simulink model "sampleModel1743_4_sub_sub"  (R2023a)
settings: Solver=VariableStepAuto  StartTime=0.0  StopTime=10.0  RelTol=1e-3
libraries: hdlsllib x4, simulink x2
settings Model: Creator=user1  LastModifiedBy=user1

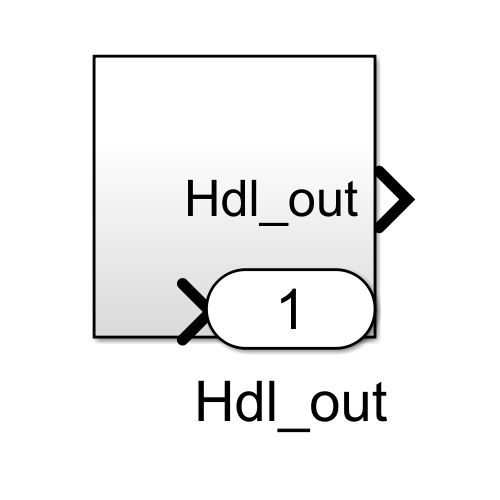
[thumbnail: Simulink's stored preview of the top-level diagram]
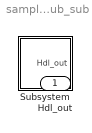
== system sampleModel1743_4_sub_sub ==
  Subsystem : Subsystem
  Hdl_out : Outport  OutDataTypeStr=uint8

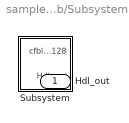
== system sampleModel1743_4_sub_sub/Subsystem ==
  Subsystem : Subsystem
  Hdl_out : Outport  OutDataTypeStr=uint8

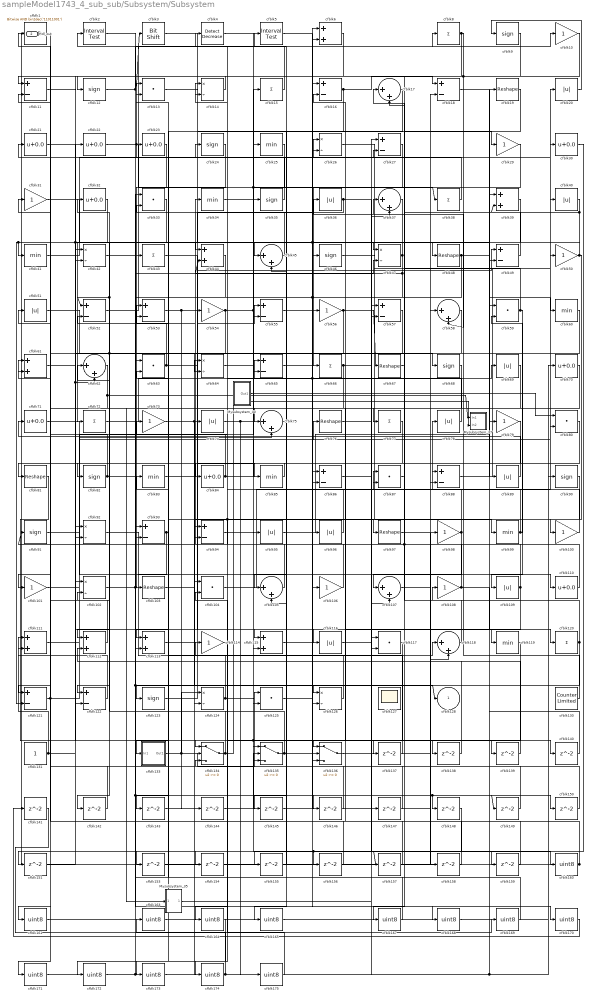
== system sampleModel1743_4_sub_sub/Subsystem/Subsystem ==
  Mysubsystem_35 : Subsystem  TreatAsAtomicUnit=on  RTWFcnName=Mysubsystem_35
      settings: RTWFcnNameOpts=User specified  RTWFileNameOpts=Use function name
  Mysubsystem_37 : Subsystem  TreatAsAtomicUnit=on  RTWFcnName=Mysubsystem_37
      settings: RTWFcnNameOpts=User specified  RTWFileNameOpts=Use function name
  Mysubsystem_40 : Subsystem  TreatAsAtomicUnit=on  RTWFcnName=Mysubsystem_40
      settings: RTWFcnNameOpts=User specified  RTWFileNameOpts=Use function name
  cfblk1 : simulink/Logic and Bit Operations/Bitwise Operator  logicop=AND  UseBitMask=on  BitMask=bin2dec('11011001')  BitMaskRealWorld=Stored Integer
      settings: LibrarySourceBlock=|
      | hdlsllib/Logic and Bit
      | Operations/Bitwise
      | Operator
  cfblk{10,29,31,50,54,56,73,79,98,100..101,106,108,114} (14 alike) : Gain  OutDataTypeStr=uint8
  cfblk{14,26,42,47,64,92,102,124,126} (9 alike) : Product  Inputs=*/  OutDataTypeStr=uint8  RndMeth=Zero  SaturateOnIntegerOverflow=on
  cfblk{19,48,67,76,81,97,103} (7 alike) : Reshape
  cfblk{13,33,59,63,80,87,104,117,125} (9 alike) : DotProduct  OutDataTypeStr=uint8
  cfblk{17,37,45,58,62,75,105,107,118} (9 alike) : Sum  Inputs=|++  OutDataTypeStr=uint8
  cfblk{20,36,40,51,69,74,78,89,95..96,109,116} (12 alike) : Abs  OutDataTypeStr=uint8  SaturateOnIntegerOverflow=off
  cfblk{11,16,18,27,49,52..53,55,57,65,86,88,93..94,121..122} (16 alike) : Sum  Inputs=+-  OutDataTypeStr=uint8
  cfblk{21..23,30,32,70..71,84,110} (9 alike) : Bias  Bias=0.0  SaturateOnIntegerOverflow=off
  cfblk{6,39,44,61,111..113,115} (8 alike) : Sum  OutDataTypeStr=uint8
  cfblk{25,34,41,60,83,85,99,119} (8 alike) : MinMax  OutDataTypeStr=uint8
  cfblk{9,12,24,35,46,68,82,90..91,123} (10 alike) : Signum
  cfblk{8,15,38,43,66,72,77,120} (8 alike) : Sum  Inputs=+  OutDataTypeStr=uint8
  cfblk127 : Scope
      settings: Floating=on
  cfblk130 : hdlsllib/Sources/Counter Limited  uplimit=7  tsamp=-1
  cfblk131 : Constant  OutDataTypeStr=uint8  SampleTime=-1
  cfblk133 : Subsystem
      settings: LibrarySourceBlock=|
      | hdlsllib/Ports &
      | Subsystems/Subsystem
  cfblk134 : Switch  OutDataTypeStr=uint8  SaturateOnIntegerOverflow=off  InputSameDT=off
  cfblk135 : Switch  OutDataTypeStr=uint8  SaturateOnIntegerOverflow=off  InputSameDT=off
  cfblk136 : Switch  OutDataTypeStr=uint8  SaturateOnIntegerOverflow=off  InputSameDT=off
  cfblk{137..151,153..159} (22 alike) : Delay  SampleTime=1
  cfblk{160..161,163..165,167..175} (14 alike) : DataTypeConversion  OutDataTypeStr=uint8  SaturateOnIntegerOverflow=off  RndMeth=Floor
  cfblk2 : hdlsllib/Logic and Bit Operations/Interval Test  IntervalClosedRight=on  uplimit=0.5  IntervalClosedLeft=on  lowlimit=-0.5  OutDataTypeStr=uint8
  cfblk3 : hdlsllib/Logic and Bit Operations/Bit Shift  mode=Shift Left Logical  N=0
  cfblk4 : simulink/Logic and Bit Operations/Detect Decrease  vinit=0.0  OutDataTypeStr=uint8
      settings: LibrarySourceBlock=|
      | hdlsllib/Logic and Bit
      | Operations/Detect
      | Decrease
  cfblk5 : hdlsllib/Logic and Bit Operations/Interval Test  IntervalClosedRight=on  uplimit=0.5  IntervalClosedLeft=on  lowlimit=-0.5  OutDataTypeStr=uint8
  cfblk128 : Outport  OutDataTypeStr=uint8  VectorParamsAs1DForOutWhenUnconnected=off
  Hdl_out : Outport  Port=2  OutDataTypeStr=uint8
  wires:
  Mysubsystem_40/1(Out1) -> cfblk80/1
  Mysubsystem_35/1(Out1) -> cfblk117/2
  cfblk70/1 -> Mysubsystem_35/1(In1)
  cfblk175/1 -> cfblk114/1
  cfblk174/1 -> cfblk79/1, cfblk90/1, cfblk163/1
  cfblk173/1 -> cfblk57/2
  cfblk148/1 -> cfblk173/1
  cfblk172/1 -> cfblk57/1
  cfblk164/1 -> cfblk172/1
  cfblk171/1 -> cfblk124/2, cfblk33/1
  cfblk170/1 -> cfblk141/1
  cfblk5/1 -> cfblk170/1
  cfblk169/1 -> cfblk63/2
  cfblk141/1 -> cfblk169/1
  cfblk168/1 -> cfblk19/1
  cfblk167/1 -> cfblk63/1
  cfblk19/1 -> cfblk167/1
  cfblk165/1 -> cfblk117/1
  cfblk119/1 -> cfblk165/1
  cfblk117/1 -> cfblk164/1
  cfblk163/1 -> cfblk70/1
  cfblk161/1 -> cfblk104/1
  cfblk1/1 -> cfblk161/1
  cfblk160/1 -> cfblk1/1, Hdl_out/1
  cfblk159/1 -> cfblk135/3
  cfblk158/1 -> cfblk26/2
  cfblk97/1 -> cfblk158/1
  cfblk157/1 -> cfblk134/3
  cfblk156/1 -> cfblk92/1
  cfblk155/1 -> cfblk45/2
  cfblk79/1 -> cfblk155/1
  cfblk154/1 -> cfblk104/2
  cfblk153/1 -> cfblk118/2
  cfblk151/1 -> cfblk42/1
  cfblk30/1 -> cfblk151/1
  cfblk150/1 -> cfblk134/2
  cfblk149/1 -> cfblk105/2
  cfblk147/1 -> cfblk11/2
  cfblk116/1 -> cfblk147/1
  cfblk146/1 -> cfblk64/1
  cfblk145/1 -> cfblk6/2
  cfblk144/1 -> cfblk88/2
  cfblk143/1 -> cfblk135/2
  cfblk142/1 -> cfblk102/1
  cfblk140/1 -> cfblk39/1
  cfblk65/1 -> cfblk140/1
  cfblk139/1 -> cfblk112/2
  cfblk86/1 -> cfblk139/1
  cfblk138/1 -> cfblk13/2
  cfblk137/1 -> cfblk94/1
  cfblk21/1 -> cfblk137/1
  cfblk135/1 -> cfblk102/2, cfblk138/1
  cfblk38/1 -> cfblk16/2
  cfblk6/1 -> cfblk92/2
  cfblk77/1 -> cfblk105/1
  cfblk25/1 -> cfblk115/2
  cfblk124/1 -> cfblk156/1, cfblk157/1, cfblk136/3, cfblk83/1
  cfblk115/1 -> cfblk86/1
  cfblk75/1 -> cfblk5/1
  cfblk37/1 -> cfblk126/2, cfblk142/1
  cfblk40/1 -> cfblk39/2, cfblk136/2
  cfblk82/1 -> cfblk31/1, cfblk47/2
  cfblk44/1 -> cfblk113/2
  cfblk56/1 -> cfblk67/1, cfblk145/1
  cfblk114/1 -> cfblk174/1
  cfblk22/1 -> cfblk96/1, cfblk23/1
  cfblk34/1 -> cfblk95/1
  cfblk61/1 -> cfblk68/1
  cfblk96/1 -> cfblk14/2
  cfblk60/1 -> cfblk82/1
  cfblk46/1 -> cfblk50/1
  cfblk104/1 -> cfblk88/1
  cfblk134/1 -> Mysubsystem_37/2(In2), cfblk32/1
  cfblk110/1 -> cfblk87/2
  cfblk50/1 -> cfblk47/1, cfblk100/1
  cfblk92/1 -> cfblk135/1
  cfblk108/1 -> cfblk120/1, cfblk61/1
  cfblk100/1 -> cfblk4/1
  cfblk2/1 -> cfblk128/1, cfblk150/1
  cfblk9/1 -> cfblk77/1
  cfblk130/1 -> cfblk36/1
  cfblk80/1 -> cfblk81/1
  cfblk39/1 -> cfblk112/1, cfblk52/1
  cfblk29/1 -> cfblk65/2
  cfblk133/1(Out1) -> cfblk125/1, cfblk124/1
  cfblk122/1 -> cfblk111/1
  cfblk58/1 -> cfblk122/1, cfblk121/1
  cfblk62/1 -> Mysubsystem_37/1(In1), cfblk122/2
  cfblk20/1 -> cfblk9/1
  cfblk109/1 -> cfblk126/1, cfblk74/1
  cfblk103/1 -> cfblk65/1
  cfblk67/1 -> cfblk27/2
  cfblk68/1 -> cfblk101/1
  cfblk36/1 -> cfblk33/2, cfblk160/1
  cfblk49/1 -> cfblk21/1
  cfblk31/1 -> cfblk53/2
  cfblk136/1 -> cfblk98/1
  cfblk18/1 -> cfblk89/1
  cfblk45/1 -> cfblk14/1
  cfblk72/1 -> cfblk6/1, cfblk58/1
  cfblk126/1 -> cfblk53/1
  cfblk95/1 -> cfblk59/1
  cfblk51/1 -> cfblk64/2
  cfblk105/1 -> cfblk94/2
  cfblk102/1 -> cfblk148/1, cfblk149/1, cfblk168/1, cfblk54/1
  cfblk118/1 -> cfblk108/1
  cfblk73/1 -> cfblk69/1, cfblk125/2
  cfblk84/1 -> cfblk62/1, cfblk80/2
  cfblk125/1 -> cfblk106/1
  cfblk57/1 -> cfblk171/1
  cfblk41/1 -> cfblk15/1
  cfblk66/1 -> cfblk113/1, cfblk37/2
  cfblk3/1 -> cfblk29/1
  cfblk94/1 -> cfblk40/1
  cfblk107/1 -> cfblk18/2
  cfblk101/1 -> cfblk76/1
  cfblk83/1 -> cfblk97/1
  cfblk98/1 -> cfblk107/1, cfblk17/2
  cfblk32/1 -> cfblk41/1, cfblk121/2, cfblk42/2
  cfblk16/1 -> cfblk18/1, cfblk143/1
  cfblk112/1 -> cfblk51/1
  cfblk74/1 -> cfblk30/1, cfblk175/1
  cfblk121/1 -> cfblk25/1, cfblk61/2
  cfblk99/1 -> cfblk78/1, cfblk59/2
  cfblk88/1 -> cfblk20/1
  cfblk90/1 -> cfblk153/1, cfblk154/1
  cfblk91/1 -> cfblk75/2
  cfblk78/1 -> cfblk24/1
  cfblk85/1 -> cfblk84/1
  cfblk63/1 -> cfblk115/1, cfblk52/2
  cfblk59/1 -> cfblk109/1, cfblk37/1
  cfblk76/1 -> cfblk27/1
  cfblk14/1 -> cfblk11/1
  cfblk24/1 -> cfblk43/1
  cfblk131/1 -> cfblk22/1, cfblk62/2, cfblk111/2
  cfblk35/1 -> cfblk13/1
  cfblk53/1 -> cfblk16/1, cfblk144/1
  cfblk87/1 -> cfblk17/1
  cfblk4/1 -> cfblk38/1, cfblk146/1
  cfblk55/1 -> cfblk46/1
  cfblk120/1 -> cfblk87/1, cfblk91/1, cfblk133/1(In1)
  cfblk10/1 -> cfblk55/2, cfblk58/2
  cfblk33/1 -> cfblk72/1
  cfblk54/1 -> cfblk26/1, cfblk159/1, cfblk93/2
  cfblk123/1 -> cfblk55/1
  cfblk42/1 -> cfblk93/1
  cfblk52/1 -> cfblk8/1
  cfblk48/1 -> cfblk123/1, cfblk86/2, cfblk60/1
  cfblk69/1 -> cfblk136/1
  cfblk12/1 -> cfblk3/1, cfblk107/2, cfblk10/1
  cfblk17/1 -> cfblk75/1
  cfblk64/1 -> cfblk35/1
  cfblk26/1 -> cfblk99/1
  cfblk71/1 -> cfblk110/1
  cfblk47/1 -> cfblk56/1, cfblk44/2, cfblk44/1
  cfblk81/1 -> cfblk134/1
  cfblk43/1 -> cfblk85/1
  cfblk106/1 -> cfblk34/1
  cfblk11/1 -> cfblk49/2, cfblk119/1
  cfblk15/1 -> cfblk2/1
  cfblk111/1 -> cfblk116/1
  cfblk23/1 -> cfblk103/1
  cfblk27/1 -> cfblk66/1
  cfblk89/1 -> cfblk71/1
  cfblk8/1 -> cfblk12/1, cfblk48/1
  cfblk93/1 -> cfblk118/1, cfblk73/1
  cfblk113/1 -> cfblk49/1
  cfblk13/1 -> cfblk45/1

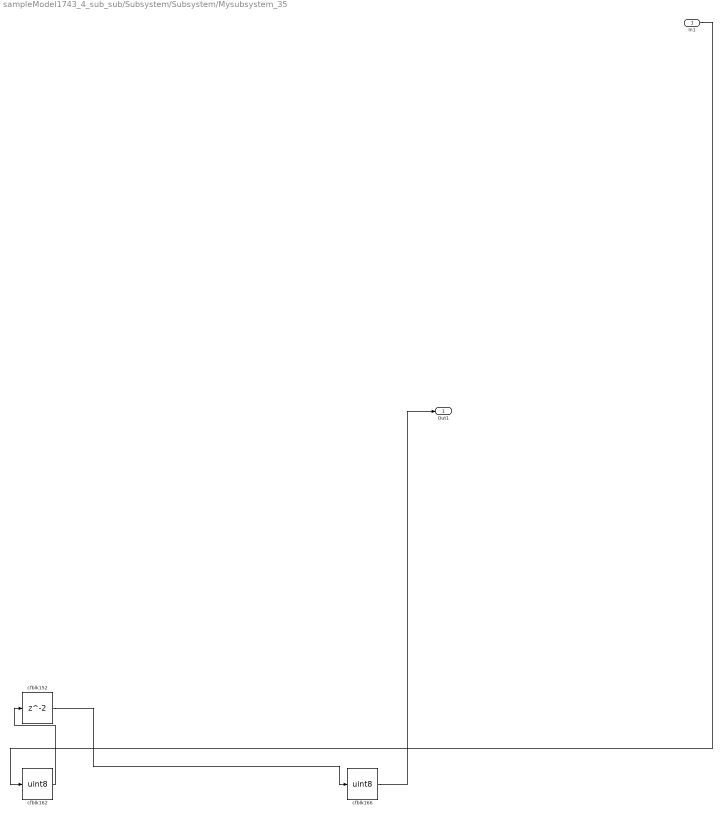
== system sampleModel1743_4_sub_sub/Subsystem/Subsystem/Mysubsystem_35 ==
  In1 : Inport
  cfblk152 : Delay  SampleTime=1
  cfblk162 : DataTypeConversion  OutDataTypeStr=uint8  SaturateOnIntegerOverflow=off  RndMeth=Floor
  cfblk166 : DataTypeConversion  OutDataTypeStr=uint8  SaturateOnIntegerOverflow=off  RndMeth=Floor
  Out1 : Outport
  wires:
  cfblk162/1 -> cfblk152/1
  In1/1 -> cfblk162/1
  cfblk152/1 -> cfblk166/1
  cfblk166/1 -> Out1/1

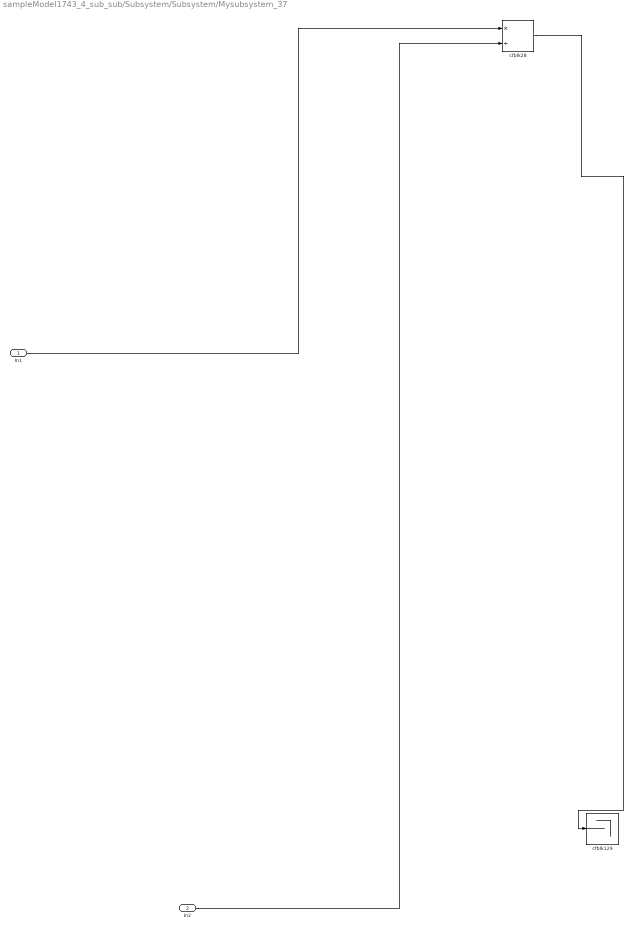
== system sampleModel1743_4_sub_sub/Subsystem/Subsystem/Mysubsystem_37 ==
  In1 : Inport
  In2 : Inport  Port=2
  cfblk129 : Terminator
  cfblk28 : Product  Inputs=*/  RndMeth=Zero  SaturateOnIntegerOverflow=on
  wires:
  cfblk28/1 -> cfblk129/1
  In2/1 -> cfblk28/2
  In1/1 -> cfblk28/1

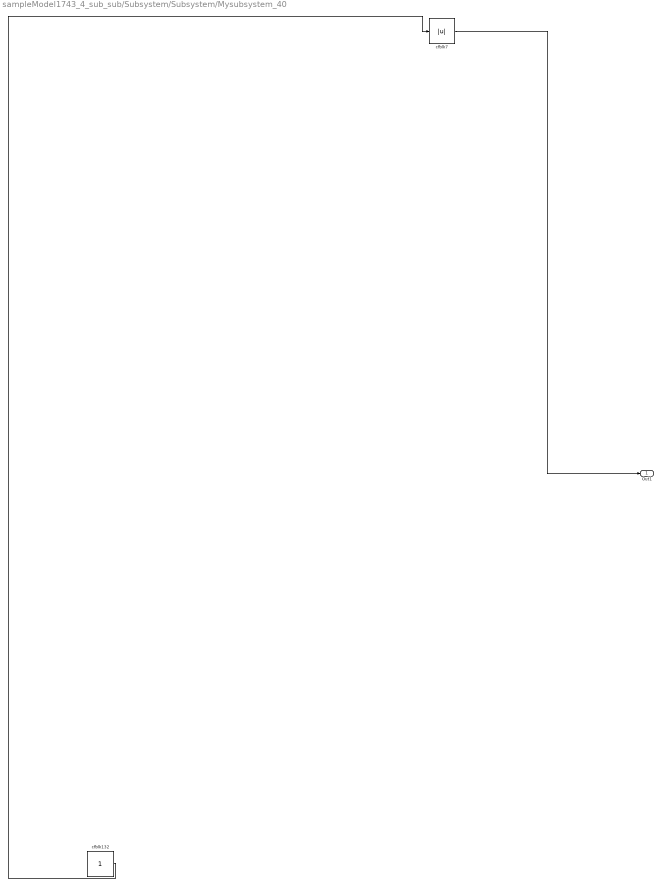
== system sampleModel1743_4_sub_sub/Subsystem/Subsystem/Mysubsystem_40 ==
  cfblk132 : Constant  SampleTime=-1
  cfblk7 : Abs  SaturateOnIntegerOverflow=off
  Out1 : Outport
  wires:
  cfblk7/1 -> Out1/1
  cfblk132/1 -> cfblk7/1

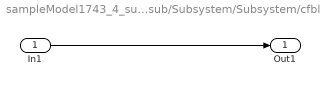
== system sampleModel1743_4_sub_sub/Subsystem/Subsystem/cfblk133 ==
  In1 : Inport
  Out1 : Outport
  wires:
  In1/1 -> Out1/1
